simulink model "Islanding_case"  (R2021b)
settings: Solver=ode3  StartTime=0.0  StopTime=2.8  FixedStep=Ts  RelTol=1e-3  EnableMultiTasking=on
InitFcn:
  | Ts=100e-6;
  | Ts_Control=100e-6;
  | Ts_Power=100e-6;
  | tvv=0.1;
  | tr=1;
  | RelayEnableTime=1;
  | En_MC=1;
  | 
  | % ================= CHOOSE THE CASE HERE ==================
  | CaseNo    = 1;      % 1 = grid connected   2 = islanding   3 = fault during islanding
  | FaultType = 'none';   % 'none'  'LG'  'LL'  'LLG'  'LLL'  'LLLG'   (not used in case 2)
  | Qmismatch = 0;      % extra capacitive reactive power (% of 1.5 MW per load); try 1 in case 2 to see the inverter trip
  | % =========================================================
  | 
  | % ---- settings derived from the case (no need to edit)
  | switch CaseNo
  |     case 1, Tisland = 100; Pmismatch = 50; Tf = 2.0;   % grid + PV supply the load, fault at 2.0 s
  |     case 2, Tisland = 2.0; Pmismatch = 0;  Tf = 100;   % breakers open at 2.0 s, no fault
  |     case 3, Tisland = 2.0; Pmismatch = 0;  Tf = 2.3;   % breakers open at 2.0 s, fault at 2.3 s
  |     otherwise, error('CaseNo must be 1, 2 or 3');
  | end
  | FaultDur = 0.1;     % fault duration (s)
  | Tf_LG   = 100; Tf_LL = 100; Tf_LLG = 100; Tf_LLL = 100; Tf_LLLG = 100;   % 100 = never
  | switch upper(FaultType)
  |     case 'LG',   Tf_LG   = Tf;
  |     case 'LL',   Tf_LL   = Tf;
  |     case 'LLG',  Tf_LLG  = Tf;
  |     case 'LLL',  Tf_LLL  = Tf;
  |     case 'LLLG', Tf_LLLG = Tf;
  |     case 'NONE'
  |     otherwise, error('FaultType must be none, LG, LL, LLG, LLL or LLLG');
  | end
undefined symbols (not defined in the file): DiscIntNeverNeededParam, Finit, Newton, Raphson, Tisland
libraries: simulink x33, spsOnDelayLib x17, powerlib_extras x11, eeGeneralControl x9, spsThreePhaseFaultLib x6, slpidlib x6, spsThreePhaseVIMeasurementLib x4, spsSampleandHoldLib x4, spsAlphaBetaZerotodq0Lib x4, spsThreePhaseSourceLib x4, spsThreePhaseBreakerLib x3, simulink_extras x3
(part 4 of 4)

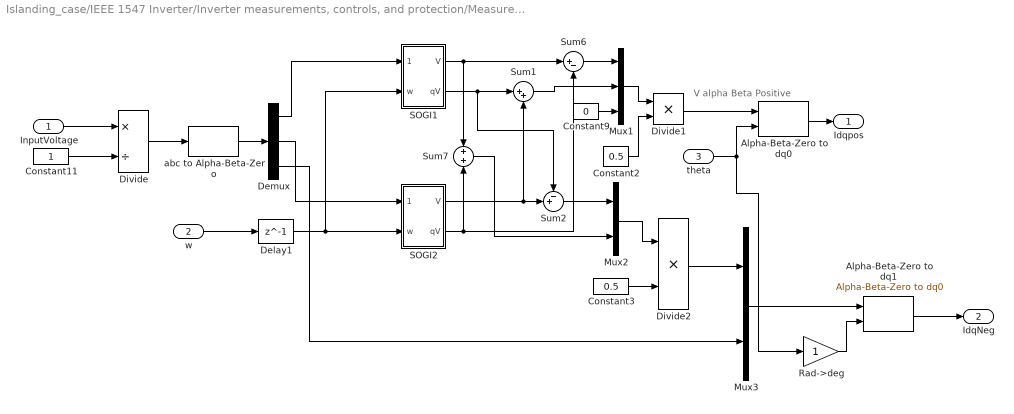
== system Islanding_case/IEEE 1547 Inverter/Inverter measurements, controls, and protection/Measurements/DSOGI PLL1 ==
  note: V alpha Beta
      | Positive
  InputVoltage : Inport
  "w " : Inport  Port=2
  theta : Inport  Port=3
  Alpha-Beta-Zero to dq0 : spsAlphaBetaZerotodq0Lib/Alpha-Beta-Zero to dq0  Alignment=Aligned with phase A axis
  Alpha-Beta-Zero to dq1 : spsAlphaBetaZerotodq0Lib/Alpha-Beta-Zero to dq0  Alignment=Aligned with phase A axis
  Constant11 : Constant
  Constant2 : Constant  Value=0.5
  Constant3 : Constant  Value=0.5
  Constant9 : Constant  Value=0
  Delay1 : Delay  DelayLength=1  InitialCondition=0
  Demux : Demux  Outputs=3
  Divide : Product  Inputs=*/
  Divide1 : Product  Inputs=**
  Divide2 : Product  Inputs=**
  Mux1 : Mux  Inputs=3
  Mux2 : Mux  Inputs=2
  Mux3 : Mux  Inputs=2
  Rad->deg : Gain
  SOGI1 : Subsystem
  SOGI2 : Subsystem
  Sum1 : Sum  Inputs=|++
  Sum2 : Sum  Inputs=-+|
  Sum6 : Sum  Inputs=|+-
  Sum7 : Sum  Inputs=+|+
  abc to Alpha-Beta-Zero : spsabctoAlphaBetaZeroLib/abc to Alpha-Beta-Zero
  Idqpos : Outport  VectorParamsAs1DForOutWhenUnconnected=off
  IdqNeg : Outport  Port=2  VectorParamsAs1DForOutWhenUnconnected=off
  wires:
  Rad->deg/1 -> Alpha-Beta-Zero to dq1/2
  theta/1 -> Alpha-Beta-Zero to dq0/2, Rad->deg/1
  Alpha-Beta-Zero to dq1/1 -> IdqNeg/1
  Constant11/1 -> Divide/2
  "w "/1 -> Delay1/1
  Divide/1 -> abc to Alpha-Beta-Zero/1
  Delay1/1 -> SOGI1/2(w), SOGI2/2(w)
  InputVoltage/1 -> Divide/1
  Sum1/1 -> Mux1/2
  Constant2/1 -> Divide1/2
  SOGI2/2(qV) -> Sum7/2, Sum6/2
  SOGI1/1(V) -> Sum7/1, Sum6/1
  Mux1/1 -> Divide1/1
  Sum2/1 -> Mux2/1
  Sum6/1 -> Mux1/1
  Divide1/1 -> Alpha-Beta-Zero to dq0/1
  Constant3/1 -> Divide2/2
  SOGI2/1(V) -> Sum2/2, Sum1/2
  Alpha-Beta-Zero to dq0/1 -> Idqpos/1
  Divide2/1 -> Mux3/1
  Mux2/1 -> Divide2/1
  Sum7/1 -> Mux2/2
  Demux/2 -> SOGI2/1(Vbeta)
  Demux/1 -> SOGI1/1(Valpha)
  Constant9/1 -> Mux1/3
  SOGI1/2(qV) -> Sum2/1, Sum1/1
  Mux3/1 -> Alpha-Beta-Zero to dq1/1
  Demux/3 -> Mux3/2
  abc to Alpha-Beta-Zero/1 -> Demux/1

== system Islanding_case/IEEE 1547 Inverter/Inverter measurements, controls, and protection/Protection /RMS1 ==
  note: Gilbert Sybille, Pierre Giroux
      | Power System Simulation Laboratory
      | IREQ, Hydro-Quebc
  note: Discrete RMS value
  In : Inport
  Freq : Inport  Port=2
  Discrete Mean value : Subsystem  AncestorBlock=|  DialogController=POWERSYS.PowerSysDialog  mask(Discrete Mean value){Ts=Ts, Vinit=Mag_Init*Mag_Init, Freq=50}
      | powerlib_extras/Discrete
      | Measurements/Discrete 
      | Mean value
      mask prompts: Ts "Sample time:"; Vinit "Initial input (DC component):"; Freq "Nominal Frequency (Hz)"
      mask help: Compute the mean value of the input signal over a running window of one cycle of the specified fundamental frequency. For the first cycle of simulation, the output is held constant to the specified initial input value.
      mask init:
      | SamplesPerCycle=1/Freq/Ts;
      | RoundSamplesPerCycle=ceil(SamplesPerCycle);
      | Delay=RoundSamplesPerCycle*Ts;
      | Corr1=(SamplesPerCycle-RoundSamplesPerCycle)/2;
      | Corr2=(SamplesPerCycle-RoundSamplesPerCycle)/SamplesPerCycle;
      | K1=Corr1*Corr2;
      | K2=Corr2 + Corr1*Corr2;
      | power_initmask();
      mask Help: This block is part of a subset of blocks in the Extras library that does not have documentation associated with it, other than the block mask description.
      mask Display: disp('Mean\n(discrete)')
  Product : Product  InputSameDT=on  SaturateOnIntegerOverflow=on  OutDataTypeStr=Inherit: Same as first input
  Saturation : Saturate  UpperLimit=Inf  LowerLimit=0
  Sqrt : Sqrt  AlgorithmType=Newton-Raphson  SaturateOnIntegerOverflow=on
  RMS : Outport  InitialOutput=0  VectorParamsAs1DForOutWhenUnconnected=off
  wires:
  Freq/1 -> Discrete Mean value/2(Freq)
  In/1 -> Product/2, Product/1
  Sqrt/1 -> RMS/1
  Product/1 -> Discrete Mean value/1(In)
  Discrete Mean value/1(Mean) -> Saturation/1
  Saturation/1 -> Sqrt/1

== system Islanding_case/IEEE 1547 Inverter/Inverter measurements, controls, and protection/Protection /RMS2 ==
  note: Gilbert Sybille, Pierre Giroux
      | Power System Simulation Laboratory
      | IREQ, Hydro-Quebc
  note: Discrete RMS value
  In : Inport
  Freq : Inport  Port=2
  Discrete Mean value : Subsystem  AncestorBlock=|  DialogController=POWERSYS.PowerSysDialog  mask(Discrete Mean value){Ts=Ts, Vinit=Mag_Init*Mag_Init, Freq=50}
      | powerlib_extras/Discrete
      | Measurements/Discrete 
      | Mean value
      mask prompts: Ts "Sample time:"; Vinit "Initial input (DC component):"; Freq "Nominal Frequency (Hz)"
      mask help: Compute the mean value of the input signal over a running window of one cycle of the specified fundamental frequency. For the first cycle of simulation, the output is held constant to the specified initial input value.
      mask init: same as Islanding_case/IEEE 1547 Inverter/Inverter measurements, controls, and protection/Protection /RMS1/Discrete Mean value
      mask Help: This block is part of a subset of blocks in the Extras library that does not have documentation associated with it, other than the block mask description.
      mask Display: disp('Mean\n(discrete)')
  Product : Product  InputSameDT=on  SaturateOnIntegerOverflow=on  OutDataTypeStr=Inherit: Same as first input
  Saturation : Saturate  UpperLimit=Inf  LowerLimit=0
  Sqrt : Sqrt  AlgorithmType=Newton-Raphson  SaturateOnIntegerOverflow=on
  RMS : Outport  InitialOutput=0  VectorParamsAs1DForOutWhenUnconnected=off
  wires:
  Freq/1 -> Discrete Mean value/2(Freq)
  In/1 -> Product/2, Product/1
  Sqrt/1 -> RMS/1
  Product/1 -> Discrete Mean value/1(In)
  Discrete Mean value/1(Mean) -> Saturation/1
  Saturation/1 -> Sqrt/1

== system Islanding_case/IEEE 1547 Inverter/Inverter measurements, controls, and protection/Inverter control in positive sequence/Controls and grid support functions block/If Action Subsystem ==
  f : Inport
  Action Port : ActionPort  ActionPortLabel=if(u1 < 59.964)
  Add : Sum  Inputs=+-
  Constant : Constant  Value=NomFreq-dbUF  SampleTime=-1
  Constant1 : Constant  Value=NomFreq*KUF  SampleTime=-1
  Divide : Product  Inputs=*/
  Pdelta : Outport  VectorParamsAs1DForOutWhenUnconnected=off
  wires:
  Divide/1 -> Pdelta/1
  Constant1/1 -> Divide/2
  Add/1 -> Divide/1
  Constant/1 -> Add/1
  [f] -> Add/2
  f/1 -> [f]

== system Islanding_case/IEEE 1547 Inverter/Inverter measurements, controls, and protection/Inverter control in positive sequence/Controls and grid support functions block/If Action Subsystem1 ==
  f : Inport
  Action Port : ActionPort  ActionPortLabel=if(u1> 50.036)
  Add : Sum  Inputs=-+
  Constant : Constant  Value=NomFreq+dbOF  SampleTime=-1
  Constant1 : Constant  Value=NomFreq*KOF  SampleTime=-1
  Divide : Product  Inputs=*/
  Pdelta : Outport  VectorParamsAs1DForOutWhenUnconnected=off
  wires:
  Constant/1 -> Add/2
  [f] -> Add/1
  Divide/1 -> Pdelta/1
  f/1 -> [f]
  Add/1 -> Divide/1
  Constant1/1 -> Divide/2

== system Islanding_case/IEEE 1547 Inverter/Inverter measurements, controls, and protection/Inverter control in positive sequence/Controls and grid support functions block/Ppre over freq ==
  f : Inport
  Ppu : Inport  Port=2
  Constant : Constant  Value=NomFreq+dbOF  SampleTime=-1
  NOT : Logic  Operator=NOT  IconShape=distinctive  AllPortsSameDT=off  OutDataTypeStr=boolean
  Relational Operator : RelationalOperator  OutDataTypeStr=boolean  RndMeth=Simplest
  Sample and Hold : spsSampleandHoldLib/Sample and Hold  ic=0  Ts=0
  Ppre : Outport  VectorParamsAs1DForOutWhenUnconnected=off
  wires:
  Relational Operator/1 -> NOT/1
  Ppu/1 -> [PpccPu]
  NOT/1 -> Sample and Hold/2
  [f] -> Relational Operator/1
  f/1 -> [f]
  Constant/1 -> Relational Operator/2
  Sample and Hold/1 -> Ppre/1
  [PpccPu] -> Sample and Hold/1

== system Islanding_case/IEEE 1547 Inverter/Inverter measurements, controls, and protection/Inverter control in positive sequence/Controls and grid support functions block/Ppre under freq ==
  f : Inport
  Ppu : Inport  Port=2
  Constant : Constant  Value=NomFreq-dbUF  SampleTime=-1
  NOT : Logic  Operator=NOT  IconShape=distinctive  AllPortsSameDT=off  OutDataTypeStr=boolean
  Relational Operator : RelationalOperator  Operator=<=  OutDataTypeStr=boolean  RndMeth=Simplest
  Sample and Hold : spsSampleandHoldLib/Sample and Hold  ic=0  Ts=0
  Ppre : Outport  VectorParamsAs1DForOutWhenUnconnected=off
  wires:
  Sample and Hold/1 -> Ppre/1
  [PpccPu] -> Sample and Hold/1
  NOT/1 -> Sample and Hold/2
  Relational Operator/1 -> NOT/1
  Constant/1 -> Relational Operator/2
  [f] -> Relational Operator/1
  Ppu/1 -> [PpccPu]
  f/1 -> [f]

== system Islanding_case/IEEE 1547 Inverter/Inverter measurements, controls, and protection/Inverter control in positive sequence/Controls and grid support functions block/RMS1 ==
  note: Gilbert Sybille, Pierre Giroux
      | Power System Simulation Laboratory
      | IREQ, Hydro-Quebc
  note: Discrete RMS value
  In : Inport
  Freq : Inport  Port=2
  Discrete Mean value : Subsystem  AncestorBlock=|  DialogController=POWERSYS.PowerSysDialog  mask(Discrete Mean value){Ts=Ts, Vinit=Mag_Init*Mag_Init, Freq=50}
      | powerlib_extras/Discrete
      | Measurements/Discrete 
      | Mean value
      mask prompts: Ts "Sample time:"; Vinit "Initial input (DC component):"; Freq "Nominal Frequency (Hz)"
      mask help: Compute the mean value of the input signal over a running window of one cycle of the specified fundamental frequency. For the first cycle of simulation, the output is held constant to the specified initial input value.
      mask init: same as Islanding_case/IEEE 1547 Inverter/Inverter measurements, controls, and protection/Protection /RMS1/Discrete Mean value
      mask Help: This block is part of a subset of blocks in the Extras library that does not have documentation associated with it, other than the block mask description.
      mask Display: disp('Mean\n(discrete)')
  Product : Product  InputSameDT=on  SaturateOnIntegerOverflow=on  OutDataTypeStr=Inherit: Same as first input
  Saturation : Saturate  UpperLimit=Inf  LowerLimit=0
  Sqrt : Sqrt  AlgorithmType=Newton-Raphson  SaturateOnIntegerOverflow=on
  RMS : Outport  InitialOutput=0  VectorParamsAs1DForOutWhenUnconnected=off
  wires:
  Freq/1 -> Discrete Mean value/2(Freq)
  In/1 -> Product/2, Product/1
  Sqrt/1 -> RMS/1
  Product/1 -> Discrete Mean value/1(In)
  Discrete Mean value/1(Mean) -> Saturation/1
  Saturation/1 -> Sqrt/1

== system Islanding_case/IEEE 1547 Inverter/Inverter measurements, controls, and protection/Inverter control in positive sequence/Controls and grid support functions block/RMS6 ==
  note: Gilbert Sybille, Pierre Giroux
      | Power System Simulation Laboratory
      | IREQ, Hydro-Quebc
  note: Discrete RMS value
  In : Inport
  Freq : Inport  Port=2
  Discrete Mean value : Subsystem  AncestorBlock=|  DialogController=POWERSYS.PowerSysDialog  mask(Discrete Mean value){Ts=Ts, Vinit=Mag_Init*Mag_Init, Freq=50}
      | powerlib_extras/Discrete
      | Measurements/Discrete 
      | Mean value
      mask prompts: Ts "Sample time:"; Vinit "Initial input (DC component):"; Freq "Nominal Frequency (Hz)"
      mask help: Compute the mean value of the input signal over a running window of one cycle of the specified fundamental frequency. For the first cycle of simulation, the output is held constant to the specified initial input value.
      mask init: same as Islanding_case/IEEE 1547 Inverter/Inverter measurements, controls, and protection/Protection /RMS1/Discrete Mean value
      mask Help: This block is part of a subset of blocks in the Extras library that does not have documentation associated with it, other than the block mask description.
      mask Display: disp('Mean\n(discrete)')
  Product : Product  InputSameDT=on  SaturateOnIntegerOverflow=on  OutDataTypeStr=Inherit: Same as first input
  Saturation : Saturate  UpperLimit=Inf  LowerLimit=0
  Sqrt : Sqrt  AlgorithmType=Newton-Raphson  SaturateOnIntegerOverflow=on
  RMS : Outport  InitialOutput=0  VectorParamsAs1DForOutWhenUnconnected=off
  wires:
  Freq/1 -> Discrete Mean value/2(Freq)
  In/1 -> Product/2, Product/1
  Sqrt/1 -> RMS/1
  Product/1 -> Discrete Mean value/1(In)
  Discrete Mean value/1(Mean) -> Saturation/1
  Saturation/1 -> Sqrt/1

== system Islanding_case/IEEE 1547 Inverter/Inverter measurements, controls, and protection/Inverter control in positive sequence/Controls and grid support functions block/RMS9 ==
  note: Gilbert Sybille, Pierre Giroux
      | Power System Simulation Laboratory
      | IREQ, Hydro-Quebc
  note: Discrete RMS value
  In : Inport
  Freq : Inport  Port=2
  Discrete Mean value : Subsystem  AncestorBlock=|  DialogController=POWERSYS.PowerSysDialog  mask(Discrete Mean value){Ts=Ts, Vinit=Mag_Init*Mag_Init, Freq=50}
      | powerlib_extras/Discrete
      | Measurements/Discrete 
      | Mean value
      mask prompts: Ts "Sample time:"; Vinit "Initial input (DC component):"; Freq "Nominal Frequency (Hz)"
      mask help: Compute the mean value of the input signal over a running window of one cycle of the specified fundamental frequency. For the first cycle of simulation, the output is held constant to the specified initial input value.
      mask init: same as Islanding_case/IEEE 1547 Inverter/Inverter measurements, controls, and protection/Protection /RMS1/Discrete Mean value
      mask Help: This block is part of a subset of blocks in the Extras library that does not have documentation associated with it, other than the block mask description.
      mask Display: disp('Mean\n(discrete)')
  Product : Product  InputSameDT=on  SaturateOnIntegerOverflow=on  OutDataTypeStr=Inherit: Same as first input
  Saturation : Saturate  UpperLimit=Inf  LowerLimit=0
  Sqrt : Sqrt  AlgorithmType=Newton-Raphson  SaturateOnIntegerOverflow=on
  RMS : Outport  InitialOutput=0  VectorParamsAs1DForOutWhenUnconnected=off
  wires:
  Freq/1 -> Discrete Mean value/2(Freq)
  In/1 -> Product/2, Product/1
  Sqrt/1 -> RMS/1
  Product/1 -> Discrete Mean value/1(In)
  Discrete Mean value/1(Mean) -> Saturation/1
  Saturation/1 -> Sqrt/1

== system Islanding_case/IEEE 1547 Inverter/Inverter measurements, controls, and protection/Inverter control in positive sequence/Controls and grid support functions block/VV controller ==
  V : Inport
  Lookup Table Dynamic : simulink/Lookup Tables/Lookup Table Dynamic  LookUpMeth=Interpolation-Use End Values  OutDataType=fixdt('double')  OutScaling=[]  OutputDataTypeScalingMode=Specify via dialog  OutDataTypeStr=fixdt('double')  DoSatur=off
  V 1,2,3,4 : Constant  Value=[V1 V2 V3 V4]
  VAR 1,2,3,4 : Constant  Value="[Q1  Q2  Q3 Q4]"
  Qref : Outport  VectorParamsAs1DForOutWhenUnconnected=off
  wires:
  Lookup Table Dynamic/1 -> Qref/1
  VAR 1,2,3,4/1 -> Lookup Table Dynamic/3
  V 1,2,3,4/1 -> Lookup Table Dynamic/2
  V/1 -> Lookup Table Dynamic/1

== system Islanding_case/IEEE 1547 Inverter/Inverter measurements, controls, and protection/Inverter control in positive sequence/Controls and grid support functions block/VW controller ==
  V : Inport
  Lookup Table Dynamic : simulink/Lookup Tables/Lookup Table Dynamic  LookUpMeth=Interpolation-Use End Values  OutDataType=fixdt('double')  OutScaling=[]  OutputDataTypeScalingMode=Specify via dialog  OutDataTypeStr=fixdt('double')  DoSatur=off
  V 1,2 : Constant  Value=[VWatt_V1 VWatt_V2]
  Watt 1,2 : Constant  Value=[VWatt_P1 VWatt_P2]
  Pref : Outport  VectorParamsAs1DForOutWhenUnconnected=off
  wires:
  Lookup Table Dynamic/1 -> Pref/1
  Watt 1,2/1 -> Lookup Table Dynamic/3
  V 1,2/1 -> Lookup Table Dynamic/2
  V/1 -> Lookup Table Dynamic/1

== system Islanding_case/IEEE 1547 Inverter/Inverter measurements, controls, and protection/Inverter control in positive sequence/abc to dq0 /LPF fo=2000Hz ==
  LPF In : Inport
  2nd-Order Filter : powerlib_extras/Discrete  Control Blocks/Discrete  2nd-Order Filter  FilterType=Lowpass  Fo=f  Zeta=0.707  Ts=Ts  Initialize=off  Vac_Init=[0 0 Finit]  Vdc_Init=Finit  PlotResponse=off  param1=[1 500 0.1]
  2nd-Order Filter1 : powerlib_extras/Discrete  Control Blocks/Discrete  2nd-Order Filter  FilterType=Lowpass  Fo=f  Zeta=0.707  Ts=Ts  Initialize=off  Vac_Init=[0 0 Finit]  Vdc_Init=Finit  PlotResponse=off  param1=[1 500 0.1]
  2nd-Order Filter2 : powerlib_extras/Discrete  Control Blocks/Discrete  2nd-Order Filter  FilterType=Lowpass  Fo=f  Zeta=0.707  Ts=Ts  Initialize=off  Vac_Init=[0 0 Finit]  Vdc_Init=Finit  PlotResponse=off  param1=[1 500 0.1]
  Demux : Demux  Outputs=3
  Mux : Mux  Inputs=3
  LPF Out : Outport  VectorParamsAs1DForOutWhenUnconnected=off
  wires:
  Demux/1 -> 2nd-Order Filter/1
  Demux/2 -> 2nd-Order Filter1/1
  Demux/3 -> 2nd-Order Filter2/1
  LPF In/1 -> Demux/1
  Mux/1 -> LPF Out/1
  2nd-Order Filter1/1 -> Mux/2
  2nd-Order Filter/1 -> Mux/1
  2nd-Order Filter2/1 -> Mux/3

== system Islanding_case/IEEE 1547 Inverter/Inverter measurements, controls, and protection/Inverter control in positive sequence/abc to dq0 /LPF fo=60Hz ==
  LPF In : Inport
  2nd-Order Filter : powerlib_extras/Discrete  Control Blocks/Discrete  2nd-Order Filter  FilterType=Lowpass  Fo=f  Zeta=0.707  Ts=Ts  Initialize=off  Vac_Init=[0 0 Finit]  Vdc_Init=Finit  PlotResponse=off  param1=[1 500 0.1]
  2nd-Order Filter1 : powerlib_extras/Discrete  Control Blocks/Discrete  2nd-Order Filter  FilterType=Lowpass  Fo=f  Zeta=0.707  Ts=Ts  Initialize=off  Vac_Init=[0 0 Finit]  Vdc_Init=Finit  PlotResponse=off  param1=[1 500 0.1]
  2nd-Order Filter2 : powerlib_extras/Discrete  Control Blocks/Discrete  2nd-Order Filter  FilterType=Lowpass  Fo=f  Zeta=0.707  Ts=Ts  Initialize=off  Vac_Init=[0 0 Finit]  Vdc_Init=Finit  PlotResponse=off  param1=[1 500 0.1]
  Demux : Demux  Outputs=3
  Mux : Mux  Inputs=3
  LPF Out : Outport  VectorParamsAs1DForOutWhenUnconnected=off
  wires:
  2nd-Order Filter2/1 -> Mux/3
  2nd-Order Filter/1 -> Mux/1
  2nd-Order Filter1/1 -> Mux/2
  Mux/1 -> LPF Out/1
  LPF In/1 -> Demux/1
  Demux/3 -> 2nd-Order Filter2/1
  Demux/2 -> 2nd-Order Filter1/1
  Demux/1 -> 2nd-Order Filter/1

== system Islanding_case/IEEE 1547 Inverter/Inverter measurements, controls, and protection/Measurements/DSOGI PLL/PI ==
  Set : Inport
  FeedBack : Inport  Port=2
  Constant7 : Constant  Value=66.64
  Constant8 : Constant  Value=2207
  Discrete-Time Integrator1 : DiscreteIntegrator  InitialCondition=2*pi*NomFreq  SampleTime=-1  LimitOutput=on  UpperSaturationLimit=439  LowerSaturationLimit=0  ICPrevOutput=DiscIntNeverNeededParam  ICPrevScaledInput=DiscIntNeverNeededParam
  Product : Product
  Product1 : Product
  Saturation : Saturate  UpperLimit=439.8  LowerLimit=0
  Sum6 : Sum  Inputs=|+-
  Sum7 : Sum  Inputs=|++
  Out : Outport  VectorParamsAs1DForOutWhenUnconnected=off
  wires:
  Discrete-Time Integrator1/1 -> Sum7/2
  Saturation/1 -> Out/1
  Constant8/1 -> Product1/2
  Set/1 -> Sum6/1
  Sum7/1 -> Saturation/1
  Product/1 -> Sum7/1
  Constant7/1 -> Product/1
  Sum6/1 -> Product1/1, Product/2
  FeedBack/1 -> Sum6/2
  Product1/1 -> Discrete-Time Integrator1/1

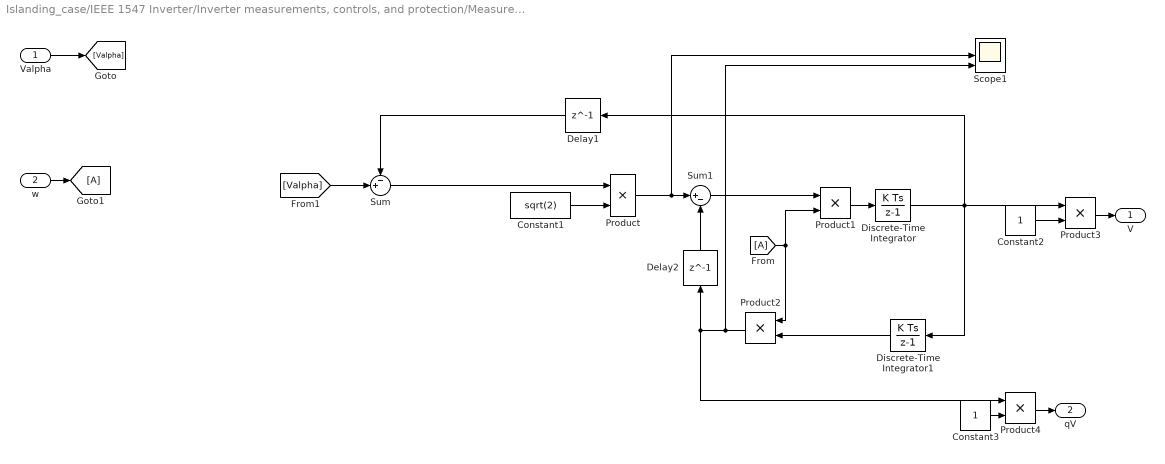
== system Islanding_case/IEEE 1547 Inverter/Inverter measurements, controls, and protection/Measurements/DSOGI PLL/SOGI1 ==
  Valpha : Inport
  w : Inport  Port=2
  Constant1 : Constant  Value=sqrt(2)
  Constant2 : Constant
  Constant3 : Constant
  Delay1 : Delay  DelayLength=1  InitialCondition=0
  Delay2 : Delay  DelayLength=1  InitialCondition=0
  Discrete-Time Integrator : DiscreteIntegrator  SampleTime=-1  ICPrevOutput=DiscIntNeverNeededParam  ICPrevScaledInput=DiscIntNeverNeededParam
  Discrete-Time Integrator1 : DiscreteIntegrator  SampleTime=-1  ICPrevOutput=DiscIntNeverNeededParam  ICPrevScaledInput=DiscIntNeverNeededParam
  Product{,1..4} (5 alike) : Product
  Scope1 : Scope  NumInputPorts=3
  Sum : Sum  Inputs=-+|
  Sum1 : Sum  Inputs=|+-
  V : Outport  VectorParamsAs1DForOutWhenUnconnected=off
  qV : Outport  Port=2  VectorParamsAs1DForOutWhenUnconnected=off
  wires:
  Delay1/1 -> Sum/1
  [Valpha] -> Sum/2
  Constant1/1 -> Product/2
  Delay2/1 -> Sum1/2
  Sum/1 -> Product/1
  Product/1 -> Scope1/2, Sum1/1
  Product1/1 -> Discrete-Time Integrator/1
  Discrete-Time Integrator/1 -> Discrete-Time Integrator1/1, Delay1/1, Product3/1
  Discrete-Time Integrator1/1 -> Product2/2
  Constant2/1 -> Product3/2
  Sum1/1 -> Product1/1
  Constant3/1 -> Product4/2
  [A] -> Product1/2, Product2/1
  Product4/1 -> qV/1
  Product3/1 -> V/1
  Valpha/1 -> [Valpha]
  w/1 -> [A]
  Product2/1 -> Scope1/3, Product4/1, Delay2/1

== system Islanding_case/IEEE 1547 Inverter/Inverter measurements, controls, and protection/Measurements/DSOGI PLL/SOGI2 ==
  Vbeta : Inport
  w : Inport  Port=2
  Constant1 : Constant  Value=sqrt(2)
  Constant2 : Constant
  Constant3 : Constant
  Delay1 : Delay  DelayLength=1  InitialCondition=0
  Delay2 : Delay  DelayLength=1  InitialCondition=0
  Discrete-Time Integrator : DiscreteIntegrator  SampleTime=-1  ICPrevOutput=DiscIntNeverNeededParam  ICPrevScaledInput=DiscIntNeverNeededParam
  Discrete-Time Integrator1 : DiscreteIntegrator  SampleTime=-1  ICPrevOutput=DiscIntNeverNeededParam  ICPrevScaledInput=DiscIntNeverNeededParam
  Product{,1..4} (5 alike) : Product
  Sum : Sum  Inputs=-+|
  Sum1 : Sum  Inputs=|+-
  V : Outport  VectorParamsAs1DForOutWhenUnconnected=off
  qV : Outport  Port=2  VectorParamsAs1DForOutWhenUnconnected=off
  wires:
  w/1 -> [A]
  Vbeta/1 -> [Vbeta]
  Product3/1 -> V/1
  Product4/1 -> qV/1
  [A] -> Product2/1, Product1/2
  Constant3/1 -> Product4/2
  Sum1/1 -> Product1/1
  Constant2/1 -> Product3/2
  Discrete-Time Integrator1/1 -> Product2/2
  Discrete-Time Integrator/1 -> Product3/1, Delay1/1, Discrete-Time Integrator1/1
  Product1/1 -> Discrete-Time Integrator/1
  Product/1 -> Sum1/1
  Sum/1 -> Product/1
  Delay2/1 -> Sum1/2
  Constant1/1 -> Product/2
  [Vbeta] -> Sum/2
  Delay1/1 -> Sum/1
  Product2/1 -> Delay2/1, Product4/1

== system Islanding_case/IEEE 1547 Inverter/Inverter measurements, controls, and protection/Measurements/DSOGI PLL1/SOGI1 ==
  Valpha : Inport
  w : Inport  Port=2
  Constant1 : Constant  Value=sqrt(2)
  Constant2 : Constant
  Constant3 : Constant
  Delay1 : Delay  DelayLength=1  InitialCondition=0
  Delay2 : Delay  DelayLength=1  InitialCondition=0
  Discrete-Time Integrator : DiscreteIntegrator  SampleTime=-1  ICPrevOutput=DiscIntNeverNeededParam  ICPrevScaledInput=DiscIntNeverNeededParam
  Discrete-Time Integrator1 : DiscreteIntegrator  SampleTime=-1  ICPrevOutput=DiscIntNeverNeededParam  ICPrevScaledInput=DiscIntNeverNeededParam
  Product{,1..4} (5 alike) : Product
  Scope1 : Scope  NumInputPorts=3
  Sum : Sum  Inputs=-+|
  Sum1 : Sum  Inputs=|+-
  V : Outport  VectorParamsAs1DForOutWhenUnconnected=off
  qV : Outport  Port=2  VectorParamsAs1DForOutWhenUnconnected=off
  wires:
  Delay1/1 -> Sum/1
  [Valpha] -> Sum/2
  Constant1/1 -> Product/2
  Delay2/1 -> Sum1/2
  Sum/1 -> Product/1
  Product/1 -> Scope1/2, Sum1/1
  Product1/1 -> Discrete-Time Integrator/1
  Discrete-Time Integrator/1 -> Discrete-Time Integrator1/1, Delay1/1, Product3/1
  Discrete-Time Integrator1/1 -> Product2/2
  Constant2/1 -> Product3/2
  Sum1/1 -> Product1/1
  Constant3/1 -> Product4/2
  [A] -> Product1/2, Product2/1
  Product4/1 -> qV/1
  Product3/1 -> V/1
  Valpha/1 -> [Valpha]
  w/1 -> [A]
  Product2/1 -> Scope1/3, Product4/1, Delay2/1

== system Islanding_case/IEEE 1547 Inverter/Inverter measurements, controls, and protection/Measurements/DSOGI PLL1/SOGI2 ==
  Vbeta : Inport
  w : Inport  Port=2
  Constant1 : Constant  Value=sqrt(2)
  Constant2 : Constant
  Constant3 : Constant
  Delay1 : Delay  DelayLength=1  InitialCondition=0
  Delay2 : Delay  DelayLength=1  InitialCondition=0
  Discrete-Time Integrator : DiscreteIntegrator  SampleTime=-1  ICPrevOutput=DiscIntNeverNeededParam  ICPrevScaledInput=DiscIntNeverNeededParam
  Discrete-Time Integrator1 : DiscreteIntegrator  SampleTime=-1  ICPrevOutput=DiscIntNeverNeededParam  ICPrevScaledInput=DiscIntNeverNeededParam
  Product{,1..4} (5 alike) : Product
  Sum : Sum  Inputs=-+|
  Sum1 : Sum  Inputs=|+-
  V : Outport  VectorParamsAs1DForOutWhenUnconnected=off
  qV : Outport  Port=2  VectorParamsAs1DForOutWhenUnconnected=off
  wires:
  w/1 -> [A]
  Vbeta/1 -> [Vbeta]
  Product3/1 -> V/1
  Product4/1 -> qV/1
  [A] -> Product2/1, Product1/2
  Constant3/1 -> Product4/2
  Sum1/1 -> Product1/1
  Constant2/1 -> Product3/2
  Discrete-Time Integrator1/1 -> Product2/2
  Discrete-Time Integrator/1 -> Product3/1, Delay1/1, Discrete-Time Integrator1/1
  Product1/1 -> Discrete-Time Integrator/1
  Product/1 -> Sum1/1
  Sum/1 -> Product/1
  Delay2/1 -> Sum1/2
  Constant1/1 -> Product/2
  [Vbeta] -> Sum/2
  Delay1/1 -> Sum/1
  Product2/1 -> Delay2/1, Product4/1

== system Islanding_case/IEEE 1547 Inverter/Inverter measurements, controls, and protection/Protection /RMS1/Discrete Mean value ==
  note: Discrete Mean Value
  note: Pierre Giroux, Gilbert Sybille
      | Power System Simulation Laboratory
      | IREQ, Hydro-Quebc
  In : Inport
  Freq : Inport  Port=2
  Constant : Constant  Value=Vinit  SampleTime=Ts
  Discrete Variable Transport Delay : powerlib_extras/Discrete  Control Blocks/Discrete Variable Transport Delay  MaxDelay=Delay+Ts  InitialValue=0  Ts=Ts
  Gain : Gain  Gain=K1  SaturateOnIntegerOverflow=on  OutDataTypeStr=Inherit: Same as input  ParamDataTypeStr=Inherit: Same as input
  Gain1 : Gain  Gain=K2  SaturateOnIntegerOverflow=on  OutDataTypeStr=Inherit: Same as input  ParamDataTypeStr=Inherit: Same as input
  Integ4 : DiscreteIntegrator  IntegratorMethod=Integration: Trapezoidal  SampleTime=Ts  ICPrevOutput=DiscIntNeverNeededParam  ICPrevScaledInput=DiscIntNeverNeededParam
  K1 : Constant  Value=Delay  SampleTime=Ts
  Product : Product  InputSameDT=on  SaturateOnIntegerOverflow=on  OutDataTypeStr=Inherit: Same as first input
  Step : Step  Time=1/Freq  SampleTime=Ts
  Sum1 : Sum  Inputs=+-  InputSameDT=on  SaturateOnIntegerOverflow=on  OutDataTypeStr=Inherit: Same as first input
  Sum5 : Sum  InputSameDT=on  SaturateOnIntegerOverflow=on  OutDataTypeStr=Inherit: Same as first input
  Sum7 : Sum  Inputs=-+  InputSameDT=on  SaturateOnIntegerOverflow=on  OutDataTypeStr=Inherit: Same as first input
  Switch : Switch  Threshold=0.5  InputSameDT=on
  Unit Delay : UnitDelay  SampleTime=Ts  HasFrameUpgradeWarning=on
  Mean : Outport  VectorParamsAs1DForOutWhenUnconnected=off
  wires:
  Freq/1 -> Product/2
  Sum1/1 -> Sum5/2  "Correction"
  Gain/1 -> Sum1/2
  Unit Delay/1 -> Gain/1
  Gain1/1 -> Sum1/1
  K1/1 -> Discrete Variable Transport Delay/2
  Discrete Variable Transport Delay/1 -> Sum7/1
  Switch/1 -> Mean/1
  Constant/1 -> Switch/3
  Step/1 -> Switch/2
  Sum5/1 -> Switch/1
  In/1 -> Unit Delay/1, Gain1/1, Integ4/1  "In"
  Integ4/1 -> Sum7/2, Discrete Variable Transport Delay/1
  Sum7/1 -> Product/1
  Product/1 -> Sum5/1  "Mean value"

== system Islanding_case/IEEE 1547 Inverter/Inverter measurements, controls, and protection/Protection /RMS2/Discrete Mean value ==
  note: Discrete Mean Value
  note: Pierre Giroux, Gilbert Sybille
      | Power System Simulation Laboratory
      | IREQ, Hydro-Quebc
  In : Inport
  Freq : Inport  Port=2
  Constant : Constant  Value=Vinit  SampleTime=Ts
  Discrete Variable Transport Delay : powerlib_extras/Discrete  Control Blocks/Discrete Variable Transport Delay  MaxDelay=Delay+Ts  InitialValue=0  Ts=Ts
  Gain : Gain  Gain=K1  SaturateOnIntegerOverflow=on  OutDataTypeStr=Inherit: Same as input  ParamDataTypeStr=Inherit: Same as input
  Gain1 : Gain  Gain=K2  SaturateOnIntegerOverflow=on  OutDataTypeStr=Inherit: Same as input  ParamDataTypeStr=Inherit: Same as input
  Integ4 : DiscreteIntegrator  IntegratorMethod=Integration: Trapezoidal  SampleTime=Ts  ICPrevOutput=DiscIntNeverNeededParam  ICPrevScaledInput=DiscIntNeverNeededParam
  K1 : Constant  Value=Delay  SampleTime=Ts
  Product : Product  InputSameDT=on  SaturateOnIntegerOverflow=on  OutDataTypeStr=Inherit: Same as first input
  Step : Step  Time=1/Freq  SampleTime=Ts
  Sum1 : Sum  Inputs=+-  InputSameDT=on  SaturateOnIntegerOverflow=on  OutDataTypeStr=Inherit: Same as first input
  Sum5 : Sum  InputSameDT=on  SaturateOnIntegerOverflow=on  OutDataTypeStr=Inherit: Same as first input
  Sum7 : Sum  Inputs=-+  InputSameDT=on  SaturateOnIntegerOverflow=on  OutDataTypeStr=Inherit: Same as first input
  Switch : Switch  Threshold=0.5  InputSameDT=on
  Unit Delay : UnitDelay  SampleTime=Ts  HasFrameUpgradeWarning=on
  Mean : Outport  VectorParamsAs1DForOutWhenUnconnected=off
  wires:
  Freq/1 -> Product/2
  Sum1/1 -> Sum5/2  "Correction"
  Gain/1 -> Sum1/2
  Unit Delay/1 -> Gain/1
  Gain1/1 -> Sum1/1
  K1/1 -> Discrete Variable Transport Delay/2
  Discrete Variable Transport Delay/1 -> Sum7/1
  Switch/1 -> Mean/1
  Constant/1 -> Switch/3
  Step/1 -> Switch/2
  Sum5/1 -> Switch/1
  In/1 -> Unit Delay/1, Gain1/1, Integ4/1  "In"
  Integ4/1 -> Sum7/2, Discrete Variable Transport Delay/1
  Sum7/1 -> Product/1
  Product/1 -> Sum5/1  "Mean value"

== system Islanding_case/IEEE 1547 Inverter/Inverter measurements, controls, and protection/Inverter control in positive sequence/Controls and grid support functions block/RMS1/Discrete Mean value ==
  note: Discrete Mean Value
  note: Pierre Giroux, Gilbert Sybille
      | Power System Simulation Laboratory
      | IREQ, Hydro-Quebc
  In : Inport
  Freq : Inport  Port=2
  Constant : Constant  Value=Vinit  SampleTime=Ts
  Discrete Variable Transport Delay : powerlib_extras/Discrete  Control Blocks/Discrete Variable Transport Delay  MaxDelay=Delay+Ts  InitialValue=0  Ts=Ts
  Gain : Gain  Gain=K1  SaturateOnIntegerOverflow=on  OutDataTypeStr=Inherit: Same as input  ParamDataTypeStr=Inherit: Same as input
  Gain1 : Gain  Gain=K2  SaturateOnIntegerOverflow=on  OutDataTypeStr=Inherit: Same as input  ParamDataTypeStr=Inherit: Same as input
  Integ4 : DiscreteIntegrator  IntegratorMethod=Integration: Trapezoidal  SampleTime=Ts  ICPrevOutput=DiscIntNeverNeededParam  ICPrevScaledInput=DiscIntNeverNeededParam
  K1 : Constant  Value=Delay  SampleTime=Ts
  Product : Product  InputSameDT=on  SaturateOnIntegerOverflow=on  OutDataTypeStr=Inherit: Same as first input
  Step : Step  Time=1/Freq  SampleTime=Ts
  Sum1 : Sum  Inputs=+-  InputSameDT=on  SaturateOnIntegerOverflow=on  OutDataTypeStr=Inherit: Same as first input
  Sum5 : Sum  InputSameDT=on  SaturateOnIntegerOverflow=on  OutDataTypeStr=Inherit: Same as first input
  Sum7 : Sum  Inputs=-+  InputSameDT=on  SaturateOnIntegerOverflow=on  OutDataTypeStr=Inherit: Same as first input
  Switch : Switch  Threshold=0.5  InputSameDT=on
  Unit Delay : UnitDelay  SampleTime=Ts  HasFrameUpgradeWarning=on
  Mean : Outport  VectorParamsAs1DForOutWhenUnconnected=off
  wires:
  Freq/1 -> Product/2
  Sum1/1 -> Sum5/2  "Correction"
  Gain/1 -> Sum1/2
  Unit Delay/1 -> Gain/1
  Gain1/1 -> Sum1/1
  K1/1 -> Discrete Variable Transport Delay/2
  Discrete Variable Transport Delay/1 -> Sum7/1
  Switch/1 -> Mean/1
  Constant/1 -> Switch/3
  Step/1 -> Switch/2
  Sum5/1 -> Switch/1
  In/1 -> Unit Delay/1, Gain1/1, Integ4/1  "In"
  Integ4/1 -> Sum7/2, Discrete Variable Transport Delay/1
  Sum7/1 -> Product/1
  Product/1 -> Sum5/1  "Mean value"

== system Islanding_case/IEEE 1547 Inverter/Inverter measurements, controls, and protection/Inverter control in positive sequence/Controls and grid support functions block/RMS6/Discrete Mean value ==
  note: Discrete Mean Value
  note: Pierre Giroux, Gilbert Sybille
      | Power System Simulation Laboratory
      | IREQ, Hydro-Quebc
  In : Inport
  Freq : Inport  Port=2
  Constant : Constant  Value=Vinit  SampleTime=Ts
  Discrete Variable Transport Delay : powerlib_extras/Discrete  Control Blocks/Discrete Variable Transport Delay  MaxDelay=Delay+Ts  InitialValue=0  Ts=Ts
  Gain : Gain  Gain=K1  SaturateOnIntegerOverflow=on  OutDataTypeStr=Inherit: Same as input  ParamDataTypeStr=Inherit: Same as input
  Gain1 : Gain  Gain=K2  SaturateOnIntegerOverflow=on  OutDataTypeStr=Inherit: Same as input  ParamDataTypeStr=Inherit: Same as input
  Integ4 : DiscreteIntegrator  IntegratorMethod=Integration: Trapezoidal  SampleTime=Ts  ICPrevOutput=DiscIntNeverNeededParam  ICPrevScaledInput=DiscIntNeverNeededParam
  K1 : Constant  Value=Delay  SampleTime=Ts
  Product : Product  InputSameDT=on  SaturateOnIntegerOverflow=on  OutDataTypeStr=Inherit: Same as first input
  Step : Step  Time=1/Freq  SampleTime=Ts
  Sum1 : Sum  Inputs=+-  InputSameDT=on  SaturateOnIntegerOverflow=on  OutDataTypeStr=Inherit: Same as first input
  Sum5 : Sum  InputSameDT=on  SaturateOnIntegerOverflow=on  OutDataTypeStr=Inherit: Same as first input
  Sum7 : Sum  Inputs=-+  InputSameDT=on  SaturateOnIntegerOverflow=on  OutDataTypeStr=Inherit: Same as first input
  Switch : Switch  Threshold=0.5  InputSameDT=on
  Unit Delay : UnitDelay  SampleTime=Ts  HasFrameUpgradeWarning=on
  Mean : Outport  VectorParamsAs1DForOutWhenUnconnected=off
  wires:
  Freq/1 -> Product/2
  Sum1/1 -> Sum5/2  "Correction"
  Gain/1 -> Sum1/2
  Unit Delay/1 -> Gain/1
  Gain1/1 -> Sum1/1
  K1/1 -> Discrete Variable Transport Delay/2
  Discrete Variable Transport Delay/1 -> Sum7/1
  Switch/1 -> Mean/1
  Constant/1 -> Switch/3
  Step/1 -> Switch/2
  Sum5/1 -> Switch/1
  In/1 -> Unit Delay/1, Gain1/1, Integ4/1  "In"
  Integ4/1 -> Sum7/2, Discrete Variable Transport Delay/1
  Sum7/1 -> Product/1
  Product/1 -> Sum5/1  "Mean value"

== system Islanding_case/IEEE 1547 Inverter/Inverter measurements, controls, and protection/Inverter control in positive sequence/Controls and grid support functions block/RMS9/Discrete Mean value ==
  note: Discrete Mean Value
  note: Pierre Giroux, Gilbert Sybille
      | Power System Simulation Laboratory
      | IREQ, Hydro-Quebc
  In : Inport
  Freq : Inport  Port=2
  Constant : Constant  Value=Vinit  SampleTime=Ts
  Discrete Variable Transport Delay : powerlib_extras/Discrete  Control Blocks/Discrete Variable Transport Delay  MaxDelay=Delay+Ts  InitialValue=0  Ts=Ts
  Gain : Gain  Gain=K1  SaturateOnIntegerOverflow=on  OutDataTypeStr=Inherit: Same as input  ParamDataTypeStr=Inherit: Same as input
  Gain1 : Gain  Gain=K2  SaturateOnIntegerOverflow=on  OutDataTypeStr=Inherit: Same as input  ParamDataTypeStr=Inherit: Same as input
  Integ4 : DiscreteIntegrator  IntegratorMethod=Integration: Trapezoidal  SampleTime=Ts  ICPrevOutput=DiscIntNeverNeededParam  ICPrevScaledInput=DiscIntNeverNeededParam
  K1 : Constant  Value=Delay  SampleTime=Ts
  Product : Product  InputSameDT=on  SaturateOnIntegerOverflow=on  OutDataTypeStr=Inherit: Same as first input
  Step : Step  Time=1/Freq  SampleTime=Ts
  Sum1 : Sum  Inputs=+-  InputSameDT=on  SaturateOnIntegerOverflow=on  OutDataTypeStr=Inherit: Same as first input
  Sum5 : Sum  InputSameDT=on  SaturateOnIntegerOverflow=on  OutDataTypeStr=Inherit: Same as first input
  Sum7 : Sum  Inputs=-+  InputSameDT=on  SaturateOnIntegerOverflow=on  OutDataTypeStr=Inherit: Same as first input
  Switch : Switch  Threshold=0.5  InputSameDT=on
  Unit Delay : UnitDelay  SampleTime=Ts  HasFrameUpgradeWarning=on
  Mean : Outport  VectorParamsAs1DForOutWhenUnconnected=off
  wires:
  Freq/1 -> Product/2
  Sum1/1 -> Sum5/2  "Correction"
  Gain/1 -> Sum1/2
  Unit Delay/1 -> Gain/1
  Gain1/1 -> Sum1/1
  K1/1 -> Discrete Variable Transport Delay/2
  Discrete Variable Transport Delay/1 -> Sum7/1
  Switch/1 -> Mean/1
  Constant/1 -> Switch/3
  Step/1 -> Switch/2
  Sum5/1 -> Switch/1
  In/1 -> Unit Delay/1, Gain1/1, Integ4/1  "In"
  Integ4/1 -> Sum7/2, Discrete Variable Transport Delay/1
  Sum7/1 -> Product/1
  Product/1 -> Sum5/1  "Mean value"

== matlab function Islanding_case/IEEE 1547 Inverter/Inverter measurements, controls, and protection/current limiting logic ==
  data: idposref input; idposref_lim output; iqposref input; idnegref input; iqnegref input; iqposref_lim output; idnegref_lim output; iqnegref_lim output; Ilimit input
function [idposref_lim,iqposref_lim,idnegref_lim,iqnegref_lim] = CurrentLimiting(idposref,...
                           iqposref,idnegref,iqnegref,Ilimit)

%Convert dq components to sequence components
Ipos=sqrt(idposref^2+iqposref^2);
Ineg=sqrt(idnegref^2+iqnegref^2);
%Phase difference between positive and negative sequence
delta=atan2(iqposref,idposref)+atan2(-iqnegref,idnegref);
%Sequence to phase component
Ia_1=sqrt(Ipos^2+Ineg^2+2*Ipos*Ineg*cos(delta));
Ib_1=sqrt(Ipos^2+Ineg^2+2*Ipos*Ineg*cos(delta+(2*pi/3)));
Ic_1=sqrt(Ipos^2+Ineg^2+2*Ipos*Ineg*cos(delta-(2*pi/3)));

if max([Ia_1,Ib_1,Ic_1])<= Ilimit  %directly pass the references if max phase current is below the limit
    idposref_lim=idposref;
    iqposref_lim=iqposref;
    iqnegref_lim=iqnegref;
    idnegref_lim=idnegref; 

else
    Ipos=sqrt(iqposref^2); % checking phase current magnitude assuming Idposref=0
    Ineg=sqrt(idnegref^2+iqnegref^2);
    %Phase difference between positive and negative sequence
    delta=atan2(iqposref,idposref)+atan2(-iqnegref,idnegref);
    %Sequence to phase component
    Ia=sqrt(Ipos^2+Ineg^2+2*Ipos*Ineg*cos(delta));
    Ib=sqrt(Ipos^2+Ineg^2+2*Ipos*Ineg*cos(delta+(2*pi/3)));
    Ic=sqrt(Ipos^2+Ineg^2+2*Ipos*Ineg*cos(delta-(2*pi/3)));
    if max([Ia,Ib,Ic]) >= Ilimit % if phase current still higher than limit, scale the reactive currents and set idposref_lim to zero
        lambda=Ilimit/max([Ia,Ib,Ic]); %scaling factor
        iqposref_lim=lambda*iqposref; %scaled down positive seq iqref
        iqnegref_lim=lambda*iqnegref; %scaled down negative seq iqref
        idnegref_lim=lambda*idnegref;  %scaled down negative seq idref
        idposref_lim=0;  %set pos seq active current to zero
    else % if phase current is below the limit assuming idposref=0, find the maximum idposref that can be injected without violating current limit
        iqposref_lim=iqposref;
        iqnegref_lim=iqnegref;
        idnegref_lim=idnegref;
        idposref_new=0;
        while 1
            Ipos=sqrt(idposref_new^2+iqposref^2);
            Ineg=sqrt(idnegref^2+iqnegref^2);       
            delta=atan2(iqposref,idposref_new)+atan2(-iqnegref,idnegref);
            %Sequence to phase component
            Ia=sqrt(Ipos^2+Ineg^2+2*Ipos*Ineg*cos(delta));
            Ib=sqrt(Ipos^2+Ineg^2+2*Ipos*Ineg*cos(delta+(2*pi/3)));
            Ic=sqrt(Ipos^2+Ineg^2+2*Ipos*Ineg*cos(delta-(2*pi/3)));
            if max([Ia,Ib,Ic])>= Ilimit
               break
            end
            idposref_new=idposref_new+0.01*idposref/abs(idposref);
        end
        idposref_lim=idposref_new;
    end
end

== matlab function Islanding_case/Islanding Analysis (IEEE 1547)/Clearing time check ==
  data: t input; clearing_time output; i_pu input; Tis input; pass output
function [clearing_time, pass] = fcn(t, i_pu, Tis)
% IEEE 1547-2018 clause 8.1.1: cease to energize and trip within 2 s of island formation.
% clearing_time = time from island formation until inverter current < 2% of rated (-1 = not yet).
persistent tc
if isempty(tc), tc = -1; end
if tc < 0 && t > Tis + 0.01 && i_pu < 0.02
    tc = t - Tis;
end
clearing_time = tc;
pass = double(tc > 0 && tc <= 2);

== matlab function Islanding_case/IEEE 1547 Inverter/Inverter measurements, controls, and protection/Protection /TOV protection ==
  settings: updateMethod=DISCRETE  sampleTime=Ts_Control
  data: V input; Enabled input; Ts input; trip output; tdi input; td output
function [trip,td]= fcn(V,Enabled,Ts,tdi)

if Enabled==1
    
    Va = V(1);
    Vb = V(2);
    Vc = V(3);
    td=tdi;
    trip=0;
    
    if (max([abs(Va),abs(Vb),abs(Vc)])>2)
        td=tdi+Ts;
    end
    
    if (td>0)
       trip=1;
    else
        trip=0;
    end
else
    trip=0;
    td=tdi;
end
    
end

== matlab function Islanding_case/IEEE 1547 Inverter/Inverter measurements, controls, and protection/Protection /TOV protection1 ==
  settings: updateMethod=DISCRETE  sampleTime=Ts_Control
  data: V input; Enabled input; Ts input; trip output; tdi input; td output
function [trip,td]= fcn(V,Enabled,Ts,tdi)

if Enabled==1
    
    Va = V(1);
    Vb = V(2);
    Vc = V(3);
    td=tdi;
    trip=0;
    
    if (max([abs(Va),abs(Vb),abs(Vc)])>1.7)
        td=tdi+Ts;
    end
    
    if (td>1.6e-3)
       trip=1;
    else
        trip=0;
    end
else
    trip=0;
    td=tdi;
end
    
end

== matlab function Islanding_case/IEEE 1547 Inverter/Inverter measurements, controls, and protection/Protection /TOV protection2 ==
  settings: updateMethod=DISCRETE  sampleTime=Ts_Control
  data: V input; Enabled input; Ts input; trip output; tdi input; td output
function [trip,td]= fcn(V,Enabled,Ts,tdi)

if Enabled==1
    
    Va = V(1);
    Vb = V(2);
    Vc = V(3);
    td=tdi;
    trip=0;
    
    if (max([abs(Va),abs(Vb),abs(Vc)])>1.4)
        td=tdi+Ts;
    end
    
    if (td>3e-3)
       trip=1;
    else
        trip=0;
    end
else
    trip=0;
    td=tdi;
end
    
end

== matlab function Islanding_case/IEEE 1547 Inverter/Inverter measurements, controls, and protection/Protection /TOV protection3 ==
  settings: updateMethod=DISCRETE  sampleTime=Ts_Control
  data: V input; Enabled input; Ts input; trip output; tdi input; td output
function [trip,td]= fcn(V,Enabled,Ts,tdi)

if Enabled==1
    
    Va = V(1);
    Vb = V(2);
    Vc = V(3);
    td=tdi;
    trip=0;
    
    if (max([abs(Va),abs(Vb),abs(Vc)])>1.3)
        td=tdi+Ts;
    end
    
    if (td>16e-3)
       trip=1;
    else
        trip=0;
    end
else
    trip=0;
    td=tdi;
end
    
end
